simulink model "robot_16bit"  (Simulink 7.4)
settings: Solver=FixedStepDiscrete  StartTime=0.0  StopTime=50  FixedStep=0.1  RelTol=1e-3
values from neighbouring files (symbols this model uses):
  Link1 = [pi/2, 0, pi/2, 0]    [robot_parameters.m]
  Link2 = [0, 0.404, pi/2, 0]    [robot_parameters.m]
  Link3 = [-pi/2, 0, 0, 0]    [robot_parameters.m]
  Link4 = [pi/2, 0.025, 0, 0.405]    [robot_parameters.m]
  Link5 = [pi/2, 0, pi/2, 0]    [robot_parameters.m]
  Link6 = [0, 0, pi/2, 0]    [robot_parameters.m]
  NoOfLinks = 6    [robot_parameters.m]
libraries: simulink x6, vrlib x6
(part 2 of 2)

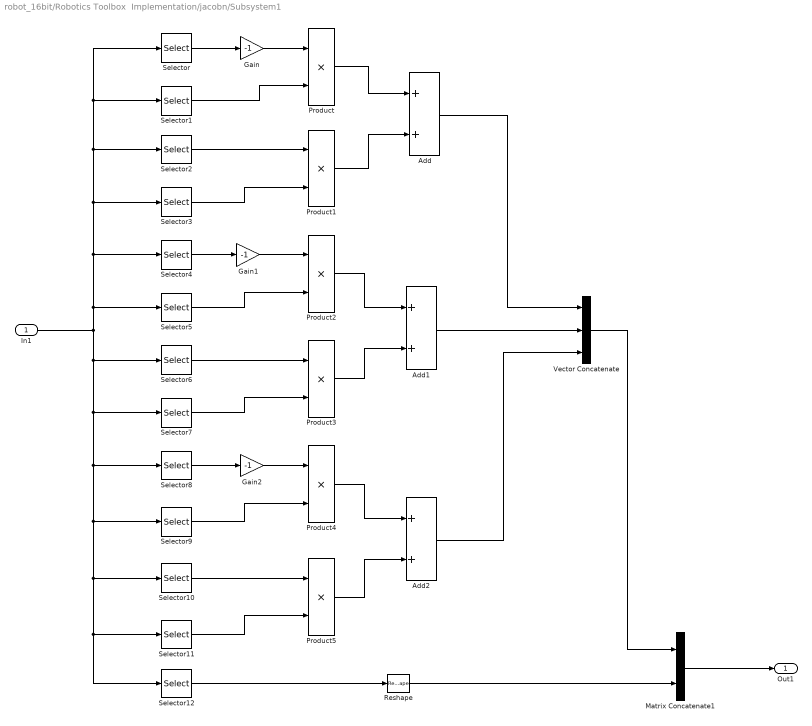
== system robot_16bit/Robotics Toolbox  Implementation/jacobn/Subsystem1 ==
  In1 : Inport
  Add : Sum  OutDataType=fixdt(1, 16)  OutScaling=2^-10
  Add1 : Sum  OutDataType=fixdt(1, 16)  OutScaling=2^-10
  Add2 : Sum  OutDataType=fixdt(1, 16)  OutScaling=2^-10
  Gain : Gain  Gain=-1  ParameterDataType=fixdt(1, 16)  ParameterScaling=2^0  OutDataType=fixdt(1, 16)  OutScaling=2^0
  Gain1 : Gain  Gain=-1  ParameterDataType=fixdt(1, 16)  ParameterScaling=2^0  OutDataType=fixdt(1, 16)  OutScaling=2^0
  Gain2 : Gain  Gain=-1  ParameterDataType=fixdt(1, 16)  ParameterScaling=2^0  OutDataType=fixdt(1, 16)  OutScaling=2^0
  Matrix Concatenate1 : Concatenate  Mode=Multidimensional array
  Product{,1..5} (6 alike) : Product  OutDataType=fixdt(1, 16)  OutScaling=2^0  RndMeth=Zero
  Reshape : Reshape  OutputDimensionality=Customize  OutputDimensions=[3,1]
  Selector : Selector  NumberOfDimensions=2  InputPortWidth=3  IndexOptions=Index vector (dialog),Index vector (dialog)  Indices=1,1  OutputSizes=1,1
  Selector1 : Selector  NumberOfDimensions=2  InputPortWidth=3  IndexOptions=Index vector (dialog),Index vector (dialog)  Indices=2,4  OutputSizes=1,1
  Selector10 : Selector  NumberOfDimensions=2  InputPortWidth=3  IndexOptions=Index vector (dialog),Index vector (dialog)  Indices=2,3  OutputSizes=1,1
  Selector11 : Selector  NumberOfDimensions=2  InputPortWidth=3  IndexOptions=Index vector (dialog),Index vector (dialog)  Indices=1,4  OutputSizes=1,1
  Selector12 : Selector  NumberOfDimensions=2  InputPortWidth=3  IndexOptions=Index vector (dialog),Index vector (dialog)  Indices=3,[1:3]  OutputSizes=1,1
  Selector2 : Selector  NumberOfDimensions=2  InputPortWidth=3  IndexOptions=Index vector (dialog),Index vector (dialog)  Indices=2,1  OutputSizes=1,1
  Selector3 : Selector  NumberOfDimensions=2  InputPortWidth=3  IndexOptions=Index vector (dialog),Index vector (dialog)  Indices=1,4  OutputSizes=1,1
  Selector4 : Selector  NumberOfDimensions=2  InputPortWidth=3  IndexOptions=Index vector (dialog),Index vector (dialog)  Indices=1,2  OutputSizes=1,1
  Selector5 : Selector  NumberOfDimensions=2  InputPortWidth=3  IndexOptions=Index vector (dialog),Index vector (dialog)  Indices=2,4  OutputSizes=1,1
  Selector6 : Selector  NumberOfDimensions=2  InputPortWidth=3  IndexOptions=Index vector (dialog),Index vector (dialog)  Indices=2,2  OutputSizes=1,1
  Selector7 : Selector  NumberOfDimensions=2  InputPortWidth=3  IndexOptions=Index vector (dialog),Index vector (dialog)  Indices=1,4  OutputSizes=1,1
  Selector8 : Selector  NumberOfDimensions=2  InputPortWidth=3  IndexOptions=Index vector (dialog),Index vector (dialog)  Indices=1,3  OutputSizes=1,1
  Selector9 : Selector  NumberOfDimensions=2  InputPortWidth=3  IndexOptions=Index vector (dialog),Index vector (dialog)  Indices=2,4  OutputSizes=1,1
  Vector Concatenate : Concatenate  NumInputs=3  Mode=Vector
  Out1 : Outport
  wires:
  Selector/1 -> Gain/1
  In1/1 -> Selector/1, Selector1/1, Selector2/1, Selector3/1, Selector4/1, Selector5/1, Selector10/1, Selector11/1, Selector12/1, Selector9/1, Selector8/1, Selector7/1, Selector6/1
  Gain/1 -> Product/1
  Selector1/1 -> Product/2
  Selector2/1 -> Product1/1
  Selector3/1 -> Product1/2
  Selector4/1 -> Gain1/1
  Gain1/1 -> Product2/1
  Selector5/1 -> Product2/2
  Selector6/1 -> Product3/1
  Selector7/1 -> Product3/2
  Selector8/1 -> Gain2/1
  Gain2/1 -> Product4/1
  Selector9/1 -> Product4/2
  Selector10/1 -> Product5/1
  Selector11/1 -> Product5/2
  Product/1 -> Add/1
  Product1/1 -> Add/2
  Product2/1 -> Add1/1
  Product3/1 -> Add1/2
  Product4/1 -> Add2/1
  Product5/1 -> Add2/2
  Add/1 -> Vector Concatenate/1
  Add1/1 -> Vector Concatenate/2
  Add2/1 -> Vector Concatenate/3
  Vector Concatenate/1 -> Matrix Concatenate1/1
  Selector12/1 -> Reshape/1
  Matrix Concatenate1/1 -> Out1/1
  Reshape/1 -> Matrix Concatenate1/2

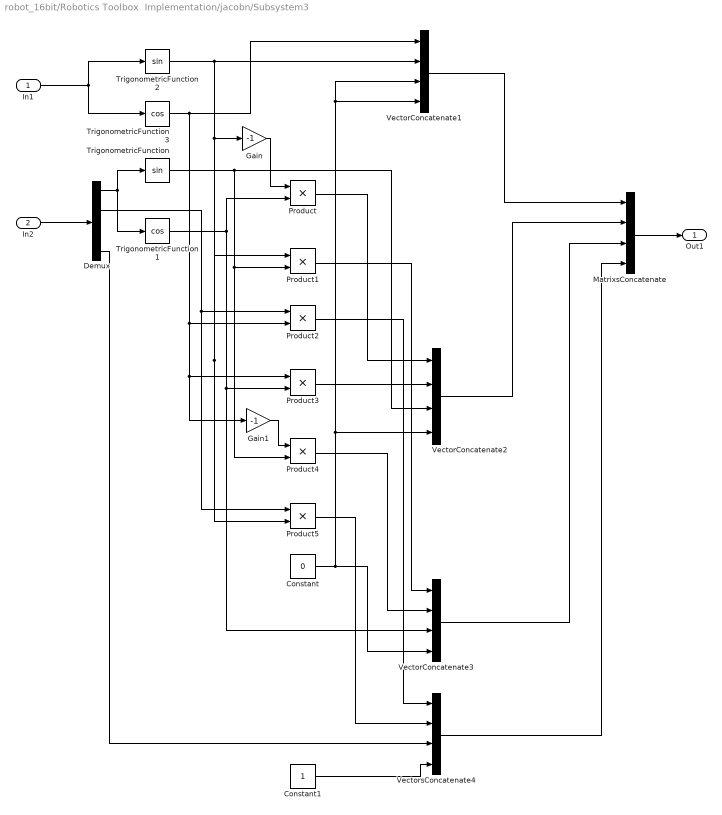
== system robot_16bit/Robotics Toolbox  Implementation/jacobn/Subsystem3 ==
  In1 : Inport  OutDataType=fixdt(1, 16)  OutScaling=2^0
  In2 : Inport  Port=2  OutDataType=fixdt(1, 16)  OutScaling=2^0
  Constant : Constant  Value=0  OutDataType=fixdt(1, 16)  OutScaling=2^0
  Constant1 : Constant  OutDataType=fixdt(1, 16)  OutScaling=2^0
  Demux : Demux
  Gain : Gain  Gain=-1  ParameterDataType=fixdt(1, 16)  ParameterScaling=2^0  OutDataType=fixdt(1, 16)  OutScaling=2^0
  Gain1 : Gain  Gain=-1  ParameterDataType=fixdt(1, 16)  ParameterScaling=2^0  OutDataType=fixdt(1, 16)  OutScaling=2^0
  MatrixsConcatenate : Concatenate  NumInputs=4  Mode=Multidimensional array  ConcatenateDimension=2
  Product{,1..5} (6 alike) : Product  OutDataType=fixdt(1, 16)  OutScaling=2^0  RndMeth=Zero
  TrigonometricFunction : Trigonometry
  TrigonometricFunction1 : Trigonometry  Operator=cos
  TrigonometricFunction2 : Trigonometry
  TrigonometricFunction3 : Trigonometry  Operator=cos
  VectorConcatenate1 : Concatenate  NumInputs=4  Mode=Vector  ConcatenateDimension=2
  VectorConcatenate2 : Concatenate  NumInputs=4  Mode=Vector  ConcatenateDimension=2
  VectorConcatenate3 : Concatenate  NumInputs=4  Mode=Vector  ConcatenateDimension=2
  VectorsConcatenate4 : Concatenate  NumInputs=4  Mode=Vector  ConcatenateDimension=2
  Out1 : Outport  OutDataType=fixdt(1, 16)  OutScaling=2^0
  wires:
  VectorsConcatenate4/1 -> MatrixsConcatenate/4
  VectorConcatenate3/1 -> MatrixsConcatenate/3
  VectorConcatenate2/1 -> MatrixsConcatenate/2
  VectorConcatenate1/1 -> MatrixsConcatenate/1
  MatrixsConcatenate/1 -> Out1/1
  Constant1/1 -> VectorsConcatenate4/4
  Constant/1 -> VectorConcatenate1/3, VectorConcatenate1/4, VectorConcatenate2/4, VectorConcatenate3/4
  Gain1/1 -> Product4/1
  Product3/1 -> VectorConcatenate2/2
  Demux/2 -> Product5/1, Product2/1
  TrigonometricFunction/1 -> Product1/2, Product4/2, VectorConcatenate2/3
  TrigonometricFunction3/1 -> VectorConcatenate1/1, Gain1/1, Product3/1, Product2/2
  TrigonometricFunction1/1 -> VectorConcatenate3/3, Product3/2, Product/2
  Gain/1 -> Product/1
  TrigonometricFunction2/1 -> Product1/1, Product5/2, Gain/1, VectorConcatenate1/2
  Demux/1 -> TrigonometricFunction1/1, TrigonometricFunction/1
  In1/1 -> TrigonometricFunction3/1, TrigonometricFunction2/1
  In2/1 -> Demux/1
  Product/1 -> VectorConcatenate2/1
  Product4/1 -> VectorConcatenate3/2
  Product1/1 -> VectorConcatenate3/1
  Product2/1 -> VectorsConcatenate4/1
  Product5/1 -> VectorsConcatenate4/2
  Demux/4 -> VectorsConcatenate4/3

== system robot_16bit/Robotics Toolbox  Implementation/jacobn/Switch Case Action Subsystem ==
  In1 : Inport  OutDataType=fixdt(1, 16)  OutScaling=2^0
  Action Port : ActionPort  ActionType=case
  Matrix Concatenate : Concatenate  NumInputs=1  Mode=Multidimensional array  ConcatenateDimension=2
  Out1 : Outport  OutDataType=fixdt(1, 16)  OutScaling=2^0
  wires:
  In1/1 -> Matrix Concatenate/1
  Matrix Concatenate/1 -> Out1/1

== system robot_16bit/Robotics Toolbox  Implementation/jacobn/Switch Case Action Subsystem1 ==
  In1 : Inport  OutDataType=fixdt(1, 16)  OutScaling=2^0
  In2 : Inport  Port=2  OutDataType=fixdt(1, 16)  OutScaling=2^0
  Action Port : ActionPort  ActionType=case
  Matrix Concatenate : Concatenate  Mode=Multidimensional array  ConcatenateDimension=2
  Out1 : Outport  OutDataType=fixdt(1, 16)  OutScaling=2^0
  wires:
  In1/1 -> Matrix Concatenate/1
  In2/1 -> Matrix Concatenate/2
  Matrix Concatenate/1 -> Out1/1

== system robot_16bit/Robotics Toolbox  Implementation/jacobn/Switch Case Action Subsystem2 ==
  In1 : Inport  OutDataType=fixdt(1, 16)  OutScaling=2^0
  In2 : Inport  Port=2  OutDataType=fixdt(1, 16)  OutScaling=2^0
  Action Port : ActionPort  ActionType=case
  Matrix Concatenate : Concatenate  Mode=Multidimensional array  ConcatenateDimension=2
  Out1 : Outport  OutDataType=fixdt(1, 16)  OutScaling=2^0
  wires:
  Matrix Concatenate/1 -> Out1/1
  In2/1 -> Matrix Concatenate/2
  In1/1 -> Matrix Concatenate/1

== system robot_16bit/Robotics Toolbox  Implementation/jacobn/Switch Case Action Subsystem3 ==
  In1 : Inport  OutDataType=fixdt(1, 16)  OutScaling=2^0
  In2 : Inport  Port=2  OutDataType=fixdt(1, 16)  OutScaling=2^0
  Action Port : ActionPort  ActionType=case
  Matrix Concatenate : Concatenate  Mode=Multidimensional array  ConcatenateDimension=2
  Out1 : Outport  OutDataType=fixdt(1, 16)  OutScaling=2^0
  wires:
  In1/1 -> Matrix Concatenate/1
  In2/1 -> Matrix Concatenate/2
  Matrix Concatenate/1 -> Out1/1

== system robot_16bit/Robotics Toolbox  Implementation/jacobn/Switch Case Action Subsystem4 ==
  In1 : Inport  OutDataType=fixdt(1, 16)  OutScaling=2^0
  In2 : Inport  Port=2  OutDataType=fixdt(1, 16)  OutScaling=2^0
  Action Port : ActionPort  ActionType=case
  Matrix Concatenate : Concatenate  Mode=Multidimensional array  ConcatenateDimension=2
  Out1 : Outport  OutDataType=fixdt(1, 16)  OutScaling=2^0
  wires:
  Matrix Concatenate/1 -> Out1/1
  In2/1 -> Matrix Concatenate/2
  In1/1 -> Matrix Concatenate/1

== system robot_16bit/Robotics Toolbox  Implementation/jacobn/Switch Case Action Subsystem5 ==
  In1 : Inport  OutDataType=fixdt(1, 16)  OutScaling=2^0
  In2 : Inport  Port=2  OutDataType=fixdt(1, 16)  OutScaling=2^0
  Action Port : ActionPort  ActionType=case
  Matrix Concatenate : Concatenate  Mode=Multidimensional array  ConcatenateDimension=2
  Out1 : Outport  OutDataType=fixdt(1, 16)  OutScaling=2^0
  wires:
  In1/1 -> Matrix Concatenate/1
  In2/1 -> Matrix Concatenate/2
  Matrix Concatenate/1 -> Out1/1

== system robot_16bit/ModelRob Implementation/Subsystem2/rpy2T1/Subsystem ==
  roll : Inport  OutDataType=fixdt(1, 16)  OutScaling=2^0
  Constant : Constant  OutDataTypeMode=Specify via dialog  OutDataType=fixdt(1,16,14)  ConRadixGroup=Best Precision: Vector-wise  OutDataTypeStr=fixdt(1,16,14)
  Constant1 : Constant  Value=0  OutDataTypeMode=Specify via dialog  OutDataType=fixdt(1,16,14)  ConRadixGroup=Best Precision: Vector-wise  OutDataTypeStr=fixdt(1,16,14)
  Cosine : simulink/Lookup Tables/Cosine  SystemSampleTime=-1  Formula=cos(2*pi*u)  NumDataPoints=(2^5)+1  OutputWordLength=16
  Gain : Gain  Gain=-1  ParameterDataType=fixdt(1, 16)  ParameterScaling=2^0  OutDataTypeMode=Specify via dialog  OutDataType=fixdt(1,16,14)  OutDataTypeStr=fixdt(1,16,14)
  Sine : simulink/Lookup Tables/Sine  SystemSampleTime=-1  Formula=sin(2*pi*u)  NumDataPoints=(2^5)+1  OutputWordLength=16
  Vector Concatenate : Concatenate  NumInputs=3  Mode=Vector
  Vector Concatenate1 : Concatenate  NumInputs=3  Mode=Vector
  Vector Concatenate2 : Concatenate  NumInputs=3  Mode=Vector
  Vector Concatenate3 : Concatenate  NumInputs=3  Mode=Multidimensional array  ConcatenateDimension=2
  Out1 : Outport  OutDataType=fixdt(1, 16)  OutScaling=2^0
  wires:
  roll/1 -> Sine/1, Cosine/1
  Constant/1 -> Vector Concatenate/1
  Cosine/1 -> Vector Concatenate1/2, Vector Concatenate2/3
  Sine/1 -> Gain/1, Vector Concatenate1/3
  Vector Concatenate/1 -> Vector Concatenate3/1
  Vector Concatenate1/1 -> Vector Concatenate3/2
  Vector Concatenate2/1 -> Vector Concatenate3/3
  Constant1/1 -> Vector Concatenate/2, Vector Concatenate/3, Vector Concatenate1/1, Vector Concatenate2/1
  Gain/1 -> Vector Concatenate2/2
  Vector Concatenate3/1 -> Out1/1

== system robot_16bit/ModelRob Implementation/Subsystem2/rpy2T1/Subsystem1 ==
  roll : Inport  OutDataType=fixdt(1, 16)  OutScaling=2^0
  Constant : Constant  OutDataTypeMode=Specify via dialog  OutDataType=fixdt(1,16,14)  ConRadixGroup=Best Precision: Vector-wise  OutDataTypeStr=fixdt(1,16,14)
  Constant1 : Constant  Value=0  OutDataTypeMode=Specify via dialog  OutDataType=fixdt(1,16,14)  ConRadixGroup=Best Precision: Vector-wise  OutDataTypeStr=fixdt(1,16,14)
  Cosine : simulink/Lookup Tables/Cosine  SystemSampleTime=-1  Formula=cos(2*pi*u)  NumDataPoints=(2^5)+1  OutputWordLength=16
      link override Cosine: OutputWordLength=16
  Gain : Gain  Gain=-1  ParameterDataType=fixdt(1, 16)  ParameterScaling=2^0  OutDataTypeMode=Specify via dialog  OutDataType=fixdt(1,16,14)  OutDataTypeStr=fixdt(1,16,14)
  Sine : simulink/Lookup Tables/Sine  SystemSampleTime=-1  Formula=sin(2*pi*u)  NumDataPoints=(2^5)+1  OutputWordLength=16
  Vector Concatenate : Concatenate  NumInputs=3  Mode=Vector
  Vector Concatenate1 : Concatenate  NumInputs=3  Mode=Vector
  Vector Concatenate2 : Concatenate  NumInputs=3  Mode=Vector
  Vector Concatenate3 : Concatenate  NumInputs=3  Mode=Multidimensional array  ConcatenateDimension=2
  Out1 : Outport  OutDataType=fixdt(1, 16)  OutScaling=2^0
  wires:
  roll/1 -> Sine/1, Cosine/1
  Vector Concatenate/1 -> Vector Concatenate3/1
  Vector Concatenate1/1 -> Vector Concatenate3/2
  Vector Concatenate2/1 -> Vector Concatenate3/3
  Cosine/1 -> Vector Concatenate/1, Vector Concatenate2/3
  Constant1/1 -> Vector Concatenate2/2, Vector Concatenate/2, Vector Concatenate1/1, Vector Concatenate1/3
  Sine/1 -> Gain/1, Vector Concatenate2/1
  Constant/1 -> Vector Concatenate1/2
  Gain/1 -> Vector Concatenate/3
  Vector Concatenate3/1 -> Out1/1

== system robot_16bit/ModelRob Implementation/Subsystem2/rpy2T1/Subsystem2 ==
  roll : Inport  OutDataType=fixdt(1, 16)  OutScaling=2^0
  Constant : Constant  OutDataTypeMode=Specify via dialog  OutDataType=fixdt(1,16,14)  ConRadixGroup=Best Precision: Vector-wise  OutDataTypeStr=fixdt(1,16,14)
  Constant1 : Constant  Value=0  OutDataTypeMode=Specify via dialog  OutDataType=fixdt(1,16,14)  ConRadixGroup=Best Precision: Vector-wise  OutDataTypeStr=fixdt(1,16,14)
  Cosine : simulink/Lookup Tables/Cosine  SystemSampleTime=-1  Formula=cos(2*pi*u)  NumDataPoints=(2^5)+1  OutputWordLength=16
  Gain : Gain  Gain=-1  ParameterDataType=fixdt(1, 16)  ParameterScaling=2^0  OutDataTypeMode=Specify via dialog  OutDataType=fixdt(1,16,14)  OutDataTypeStr=fixdt(1,16,14)
  Sine : simulink/Lookup Tables/Sine  SystemSampleTime=-1  Formula=sin(2*pi*u)  NumDataPoints=(2^5)+1  OutputWordLength=16
  Vector Concatenate : Concatenate  NumInputs=3  Mode=Vector
  Vector Concatenate1 : Concatenate  NumInputs=3  Mode=Vector
  Vector Concatenate2 : Concatenate  NumInputs=3  Mode=Vector
  Vector Concatenate3 : Concatenate  NumInputs=3  Mode=Multidimensional array  ConcatenateDimension=2
  Out1 : Outport  OutDataType=fixdt(1, 16)  OutScaling=2^0
  wires:
  roll/1 -> Sine/1, Cosine/1
  Vector Concatenate/1 -> Vector Concatenate3/1
  Vector Concatenate1/1 -> Vector Concatenate3/2
  Vector Concatenate2/1 -> Vector Concatenate3/3
  Cosine/1 -> Vector Concatenate/1, Vector Concatenate1/2
  Sine/1 -> Vector Concatenate/2, Gain/1
  Constant1/1 -> Vector Concatenate/3, Vector Concatenate1/3, Vector Concatenate2/1, Vector Concatenate2/2
  Constant/1 -> Vector Concatenate2/3
  Gain/1 -> Vector Concatenate1/1
  Vector Concatenate3/1 -> Out1/1

== system robot_16bit/Robotics Toolbox  Implementation/Subsystem1/rpy2T/Subsystem ==
  roll : Inport  OutDataType=fixdt(1, 16)  OutScaling=2^0
  Constant : Constant  OutDataType=fixdt(1, 16)  OutScaling=2^0
  Constant1 : Constant  Value=0  OutDataType=fixdt(1, 16)  OutScaling=2^0
  Gain : Gain  Gain=-1  ParameterDataType=fixdt(1, 16)  ParameterScaling=2^0  OutDataType=fixdt(1, 16)  OutScaling=2^0
  Trigonometric Function : Trigonometry
  Trigonometric Function1 : Trigonometry  Operator=cos
  Vector Concatenate : Concatenate  NumInputs=3  Mode=Vector
  Vector Concatenate1 : Concatenate  NumInputs=3  Mode=Vector
  Vector Concatenate2 : Concatenate  NumInputs=3  Mode=Vector
  Vector Concatenate3 : Concatenate  NumInputs=3  Mode=Multidimensional array  ConcatenateDimension=2
  Out1 : Outport  OutDataType=fixdt(1, 16)  OutScaling=2^0
  wires:
  roll/1 -> Trigonometric Function/1, Trigonometric Function1/1
  Constant/1 -> Vector Concatenate/1
  Trigonometric Function1/1 -> Vector Concatenate1/2, Vector Concatenate2/3
  Trigonometric Function/1 -> Gain/1, Vector Concatenate1/3
  Vector Concatenate/1 -> Vector Concatenate3/1
  Vector Concatenate1/1 -> Vector Concatenate3/2
  Vector Concatenate2/1 -> Vector Concatenate3/3
  Constant1/1 -> Vector Concatenate/2, Vector Concatenate/3, Vector Concatenate1/1, Vector Concatenate2/1
  Gain/1 -> Vector Concatenate2/2
  Vector Concatenate3/1 -> Out1/1

== system robot_16bit/Robotics Toolbox  Implementation/Subsystem1/rpy2T/Subsystem1 ==
  roll : Inport  OutDataType=fixdt(1, 16)  OutScaling=2^0
  Constant : Constant  OutDataType=fixdt(1, 16)  OutScaling=2^0
  Constant1 : Constant  Value=0  OutDataType=fixdt(1, 16)  OutScaling=2^0
  Gain : Gain  Gain=-1  ParameterDataType=fixdt(1, 16)  ParameterScaling=2^0  OutDataType=fixdt(1, 16)  OutScaling=2^0
  Trigonometric Function : Trigonometry
  Trigonometric Function1 : Trigonometry  Operator=cos
  Vector Concatenate : Concatenate  NumInputs=3  Mode=Vector
  Vector Concatenate1 : Concatenate  NumInputs=3  Mode=Vector
  Vector Concatenate2 : Concatenate  NumInputs=3  Mode=Vector
  Vector Concatenate3 : Concatenate  NumInputs=3  Mode=Multidimensional array  ConcatenateDimension=2
  Out1 : Outport  OutDataType=fixdt(1, 16)  OutScaling=2^0
  wires:
  roll/1 -> Trigonometric Function/1, Trigonometric Function1/1
  Vector Concatenate/1 -> Vector Concatenate3/1
  Vector Concatenate1/1 -> Vector Concatenate3/2
  Vector Concatenate2/1 -> Vector Concatenate3/3
  Trigonometric Function1/1 -> Vector Concatenate/1, Vector Concatenate2/3
  Constant1/1 -> Vector Concatenate2/2, Vector Concatenate/2, Vector Concatenate1/1, Vector Concatenate1/3
  Trigonometric Function/1 -> Gain/1, Vector Concatenate2/1
  Constant/1 -> Vector Concatenate1/2
  Gain/1 -> Vector Concatenate/3
  Vector Concatenate3/1 -> Out1/1

== system robot_16bit/Robotics Toolbox  Implementation/Subsystem1/rpy2T/Subsystem2 ==
  roll : Inport  OutDataType=fixdt(1, 16)  OutScaling=2^0
  Constant : Constant  OutDataType=fixdt(1, 16)  OutScaling=2^0
  Constant1 : Constant  Value=0  OutDataType=fixdt(1, 16)  OutScaling=2^0
  Gain : Gain  Gain=-1  ParameterDataType=fixdt(1, 16)  ParameterScaling=2^0  OutDataType=fixdt(1, 16)  OutScaling=2^0
  Trigonometric Function : Trigonometry
  Trigonometric Function1 : Trigonometry  Operator=cos
  Vector Concatenate : Concatenate  NumInputs=3  Mode=Vector
  Vector Concatenate1 : Concatenate  NumInputs=3  Mode=Vector
  Vector Concatenate2 : Concatenate  NumInputs=3  Mode=Vector
  Vector Concatenate3 : Concatenate  NumInputs=3  Mode=Multidimensional array  ConcatenateDimension=2
  Out1 : Outport  OutDataType=fixdt(1, 16)  OutScaling=2^0
  wires:
  roll/1 -> Trigonometric Function/1, Trigonometric Function1/1
  Vector Concatenate/1 -> Vector Concatenate3/1
  Vector Concatenate1/1 -> Vector Concatenate3/2
  Vector Concatenate2/1 -> Vector Concatenate3/3
  Trigonometric Function1/1 -> Vector Concatenate/1, Vector Concatenate1/2
  Trigonometric Function/1 -> Vector Concatenate/2, Gain/1
  Constant1/1 -> Vector Concatenate/3, Vector Concatenate1/3, Vector Concatenate2/1, Vector Concatenate2/2
  Constant/1 -> Vector Concatenate2/3
  Gain/1 -> Vector Concatenate1/1
  Vector Concatenate3/1 -> Out1/1
